simulink model "rlpitch2"  (R2019b)
settings: Solver=ode45  StartTime=0.0  StopTime=200  RelTol=1e-3  EnableMultiTasking=on
undefined symbols (not defined in the file or in its folder): DiscIntNeverNeededParam, Ts
libraries: simulink x3, rllib x1
settings Model: Creator=The MathWorks, Inc.  LastModifiedBy=Adyasha
settings DataIOCC: LimitDataPoints=on  SaveFormat=Array  ReturnWorkspaceOutputs=off  SignalLoggingName=logsOut
settings OptimizationCC: ExpressionDepthLimit=2147483647  InitFltsAndDblsToZero=on  LifeSpan=inf
settings DebuggingCC: SaveWithParameterizedLinksMsg=none  UnderspecifiedInitializationDetection=Classic  MergeDetectMultiDrivingBlocksExec=none  SignalResolutionControl=TryResolveAllWithWarning  MultiTaskDSMMsg=warning  FcnCallInpInsideContextMsg=warning  AllowSymbolicDim=off  StateNameClashWarn=warning  SFUnexpectedBacktrackingDiag=warning  SFNoUnconditionalDefaultTransitionDiag=warning  SFExecutionAtInitializationDiag=none  ArithmeticOperatorsInVariantConditions=warning
settings HardwareCC: ProdBitPerPointer=32  ProdBitPerSizeT=32  ProdBitPerPtrDiffT=32  ProdLargestAtomicFloat=None  ProdIntDivRoundTo=Undefined  ProdEndianess=Unspecified  ProdWordSize=32  ProdHWDeviceType=Specified
settings ModelReferenceCC: PropagateSignalLabelsOutOfModel=off
settings SFSimCC: SimUseLocalCustomCode=off  CustomCodeUndefinedFunction=UseInterfaceOnly
settings RTWCC: RTWUseLocalCustomCode=off
settings CodeAppCC: StateflowObjectComments=on
settings GRTTargetCC: TargetFcnLib=ansi_tfl_tmw.mat  TargetLangStandard=C89/C90 (ANSI)  GeneratePreprocessorConditionals=Disable all  CombineOutputUpdateFcns=off  GRTInterface=on
settings ConfigComp: CovMetricSettings=dw  CovHtmlReporting=on  CovSaveCumulativeToWorkspaceVar=on  CovSaveSingleToWorkspaceVar=on  CovExternalEMLEnable=off

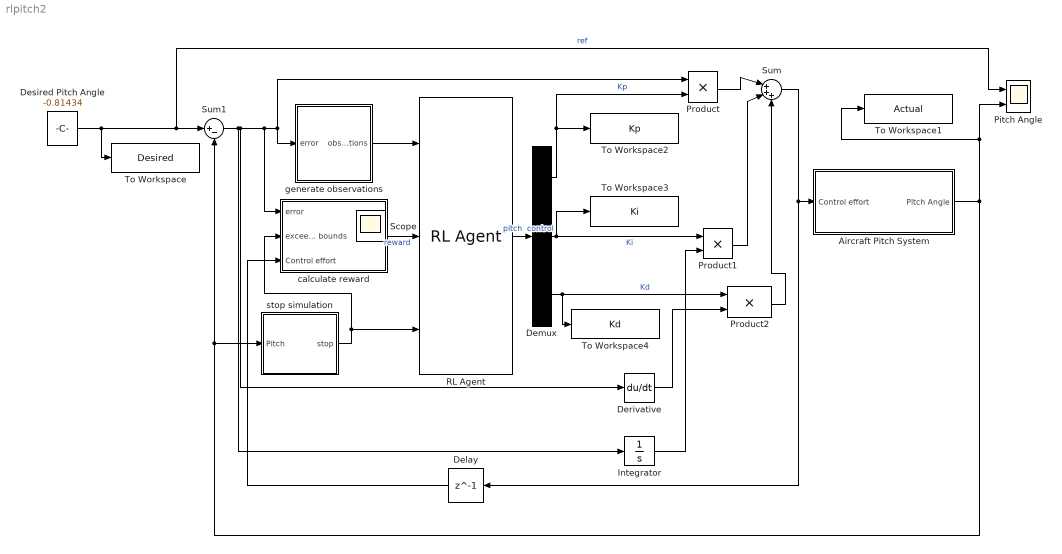
== system rlpitch2 ==
  Aircraft Pitch System : Subsystem
  Delay : Delay  DelayLength=1  InitialCondition=0
  Demux : Demux  Outputs=3
  Derivative : Derivative
  Desired Pitch Angle : Constant  Value=-0.81434
  Integrator : Integrator
  Pitch Angle : Scope  NumInputPorts=2
  Product : Product
  Product1 : Product
  Product2 : Product
  RL Agent : rllib/RL Agent  Agent=agent  ProvideReward=on  ProvideIsDone=on  ProvideCumRwd=off  TreatAsDirectFeedthrough=on  CollectLoggedSignals=on  CollectModelStates=on
      settings: SourceProductName=Reinforcement Learning Toolbox
  Sum : Sum  Inputs=|+++
  Sum1 : Sum  Inputs=|+-  SaturateOnIntegerOverflow=on
  To Workspace : ToWorkspace  VariableName=Desired  SampleTime=-1
  To Workspace1 : ToWorkspace  VariableName=Actual  SampleTime=-1
  To Workspace2 : ToWorkspace  VariableName=Kp  SaveFormat=Structure With Time  SampleTime=-1
  To Workspace3 : ToWorkspace  VariableName=Ki  SaveFormat=Structure With Time  SampleTime=-1
  To Workspace4 : ToWorkspace  VariableName=Kd  SaveFormat=Structure With Time  SampleTime=-1
  calculate reward : Subsystem
  generate observations : Subsystem
  stop simulation : Subsystem
  Scope : Scope
  wires:
  Desired Pitch Angle/1 -> Sum1/1, Pitch Angle/1, To Workspace/1  "ref"
  Sum1/1 -> Integrator/1, generate observations/1(error), Product/1, calculate reward/1(error), Derivative/1
  stop simulation/1(stop) -> RL Agent/3, calculate reward/2(exceeds bounds)
  calculate reward/1(reward) -> RL Agent/2  "reward"
  generate observations/1(observations) -> RL Agent/1
  Aircraft Pitch System/1(Pitch Angle) -> stop simulation/1(Pitch), Sum1/2, Pitch Angle/2, To Workspace1/1
  RL Agent/1 -> Demux/1  "pitch  control"
  Sum/1 -> Delay/1, Aircraft Pitch System/1(Control effort)
  Demux/1 -> Product/2, To Workspace2/1  "Kp"
  Product/1 -> Sum/1
  Integrator/1 -> Product1/2
  Product1/1 -> Sum/2
  Demux/2 -> To Workspace3/1, Product1/1  "Ki"
  Demux/3 -> Product2/1, To Workspace4/1  "Kd"
  Derivative/1 -> Product2/2
  Product2/1 -> Sum/3
  Delay/1 -> calculate reward/3(Control effort)

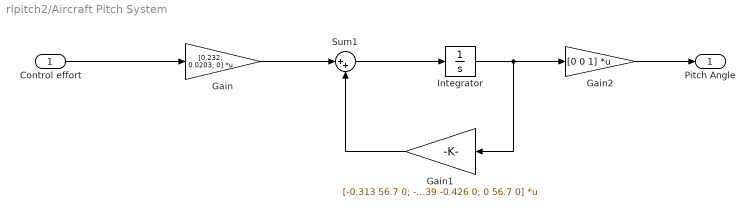
== system rlpitch2/Aircraft Pitch System ==
  Control effort : Inport
  Gain : Gain  Gain=[0.232; 0.0203; 0]  Multiplication=Matrix(K*u)
  Gain1 : Gain  Gain=[-0.313 56.7 0; -0.0139 -0.426 0; 0 56.7 0]  Multiplication=Matrix(K*u)
  Gain2 : Gain  Gain=[0 0 1]  Multiplication=Matrix(K*u)
  Integrator : Integrator
  Sum1 : Sum  Inputs=|++
  Pitch Angle : Outport  VectorParamsAs1DForOutWhenUnconnected=off
  wires:
  Gain/1 -> Sum1/1
  Sum1/1 -> Integrator/1
  Integrator/1 -> Gain1/1, Gain2/1
  Gain1/1 -> Sum1/2
  Control effort/1 -> Gain/1
  Gain2/1 -> Pitch Angle/1

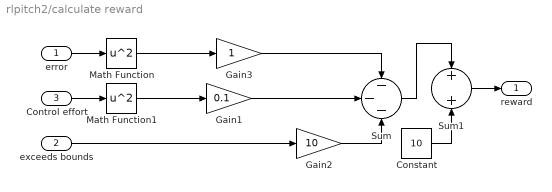
== system rlpitch2/calculate reward ==
  error : Inport
  exceeds bounds : Inport  Port=2
  Control effort : Inport  Port=3
  Constant : Constant  Value=10
  Gain1 : Gain  Gain=0.1
  Gain2 : Gain  Gain=10
  Gain3 : Gain
  Math Function : Math  Operator=square  SignedPower=off  SaturateOnIntegerOverflow=on
  Math Function1 : Math  Operator=square  SignedPower=off  SaturateOnIntegerOverflow=on
  Sum : Sum  Inputs=---  OutDataTypeStr=double
  Sum1 : Sum  OutDataTypeStr=double
  reward : Outport  VectorParamsAs1DForOutWhenUnconnected=off
  wires:
  exceeds bounds/1 -> Gain2/1
  error/1 -> Math Function/1
  Math Function/1 -> Gain3/1
  Gain3/1 -> Sum/1
  Sum/1 -> Sum1/1
  Constant/1 -> Sum1/2
  Sum1/1 -> reward/1
  Math Function1/1 -> Gain1/1
  Gain2/1 -> Sum/3
  Gain1/1 -> Sum/2
  Control effort/1 -> Math Function1/1

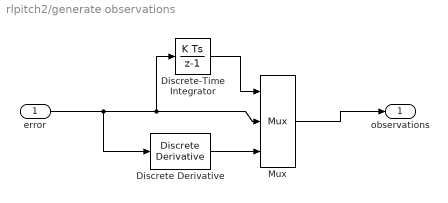
== system rlpitch2/generate observations ==
  error : Inport
  Discrete Derivative : simulink/Discrete/Discrete Derivative  gainval=1.0  ICPrevScaledInput=0.0  OutMin=[]  OutMax=[]  OutDataType=fixdt(1, 16)  OutScaling=2^-10  DoSatur=off
  Discrete-Time Integrator : DiscreteIntegrator  SampleTime=Ts  ICPrevOutput=DiscIntNeverNeededParam  ICPrevScaledInput=DiscIntNeverNeededParam
  Mux : Mux  Inputs=3
  observations : Outport  VectorParamsAs1DForOutWhenUnconnected=off
  wires:
  Discrete-Time Integrator/1 -> Mux/1
  error/1 -> Discrete Derivative/1, Discrete-Time Integrator/1, Mux/2
  Mux/1 -> observations/1
  Discrete Derivative/1 -> Mux/3

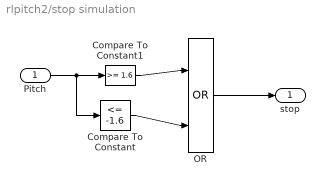
== system rlpitch2/stop simulation ==
  Pitch : Inport
  Compare To Constant : simulink/Logic and Bit Operations/Compare To Constant  relop=<=  const=-1.6  OutDataTypeStr=boolean
  Compare To Constant1 : simulink/Logic and Bit Operations/Compare To Constant  relop=>=  const=1.6  OutDataTypeStr=boolean
  OR : Logic  Operator=OR  IconShape=distinctive  AllPortsSameDT=off  OutDataTypeStr=boolean
  stop : Outport  VectorParamsAs1DForOutWhenUnconnected=off
  wires:
  Pitch/1 -> Compare To Constant/1, Compare To Constant1/1
  Compare To Constant/1 -> OR/2
  Compare To Constant1/1 -> OR/1
  OR/1 -> stop/1
